simulink model "Simu_Simulink"  (R2016a)
settings: Solver=FixedStepDiscrete  StartTime=0.0  StopTime=10  FixedStep=0.01  RelTol=1e-3
InitFcn:
  |     if ~coder.target('MATLAB')
  | coder.ceval('NMPC_Solve_initialize');
  |     end
values from neighbouring files (symbols this model uses):
  x0 = [-2; 0; 0; 0]    [NMPC_Problem_Formulation.m]    (also in Simu_Matlab.m = SIM_Plant_RK4(uOptimal(1:4,1),x0,pSimVal,Ts); Simu_Simulink_Setup.m = initData.x0)
settings Model: Creator=Deng  LastModifiedBy=idead
settings OptimizationCC: SimCompilerOptimization=on
settings HardwareCC: ProdWordSize=32  ProdHWDeviceType=Specified
settings SFSimCC: SimCustomHeaderCode="#include \"NMPC_Solve.h\""  SimCustomInitializer=NMPC_Solve_initialize();  SimCustomTerminator=NMPC_Solve_terminate();  SimUserIncludeDirs=./codegen/dll/NMPC_Solve  SimUserLibraries=NMPC_Solve.lib
settings RTWCC: GenerateReport=on  RTWUseSimCustomCode=on  CustomHeaderCode="#include \"NMPC_Solve.h\""  CustomInclude=./codegen/dll/NMPC_Solve  CustomLibrary=NMPC_Solve.lib  CustomInitializer=NMPC_Solve_initialize();  CustomTerminator=NMPC_Solve_terminate();  BuildConfiguration=Faster Runs  LaunchReport=on

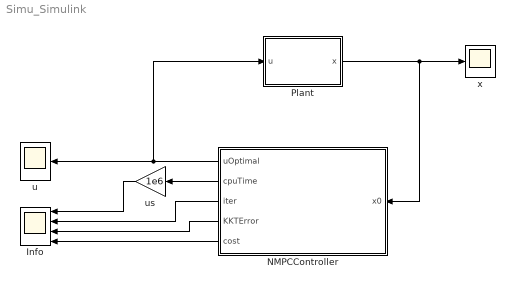
== system Simu_Simulink ==
  Info : Scope  NumInputPorts=4
  NMPCController : MATLAB Function  TreatAsAtomicUnit=on
  Plant : Subsystem
  u : Scope
  us : Gain  Gain=1e6
  x : Scope
  wires:
  NMPCController/1(uOptimal) -> Plant/1(u), u/1
  NMPCController/2(cpuTime) -> us/1
  us/1 -> Info/1
  NMPCController/3(iter) -> Info/2
  NMPCController/4(KKTError) -> Info/3
  NMPCController/5(cost) -> Info/4
  Plant/1(x) -> x/1, NMPCController/1(x0)

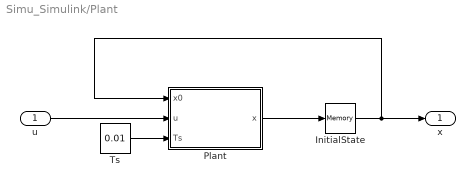
== system Simu_Simulink/Plant ==
  u : Inport
  InitialState : Memory  X0=x0
  Plant : MATLAB Function  TreatAsAtomicUnit=on
  Ts : Constant  Value=0.01
  x : Outport
  wires:
  Plant/1(x) -> InitialState/1
  InitialState/1 -> Plant/1(x0), x/1
  u/1 -> Plant/2(u)
  Ts/1 -> Plant/3(Ts)

== matlab function Simu_Simulink/Plant/Plant ==
  data: x0 input; u input; x output; Ts input
function x = plant(x0,u,Ts)
%#codegen
pSimVal = zeros(0,1);
x = SIM_Plant_RK4(u(:),x0,pSimVal,Ts);

== matlab function Simu_Simulink/NMPCController ==
  data: uOptimal output; x0 input; cpuTime output; iter output; KKTError output; cost output
function [uOptimal,cpuTime,iter,KKTError,cost]  = NMPC_Solve(x0)
%#codegen

output      = createOutput();
solution    = createNonemptySolution();

% call the generated function
coder.ceval('NMPC_Solve',...
             x0,...
             coder.wref(solution),...
             coder.wref(output));

uOptimal = solution.u(1:2,1);
cpuTime  = output.timeElapsed.total;
KKTError = output.KKTError;
iter     = output.iterTotal;
cost     = output.cost;
